simulink model "Studienarbeit"  (R2020a)
settings: Solver=VariableStepAuto  StartTime=0.0  StopTime=300  FixedStep=0.1  RelTol=1e-3
values from neighbouring files (symbols this model uses):
  driver_I = 0.1    [Buses_.mat]    (also in helperACCSetUp.m)
  driver_P = 0.2    [Buses_.mat]    (also in helperACCSetUp.m)
  initial_lane = 0    [helperACCSetUp.m]
  lr = 1.6    [Buses_.mat]    (also in helperACCSetUp.m)
  m = 1575    [Buses_.mat]    (also in helperACCSetUp.m)
  tau = 0.5    [Buses_.mat]    (also in helperACCSetUp.m)
  velocity_left_lane_max = 28    [Buses_.mat]    (also in helperManeuverSetUp.m)
  velocity_right_lane_max = 20    [Buses_.mat]    (also in helperManeuverSetUp.m)
  velocity_vehicle_B = 10    [Buses_.mat]    (also in helperManeuverSetUp.m)
  yawerr_gain = 2    [Buses_.mat]    (also in helperACCSetUp.m)
undefined symbols (not defined in the file or in its folder): Curvature, CurvatureDerivative, driving, HeadingAngle, LateralOffset, Left, Right, Strength
libraries: drivingscenarioandsensors x3, simulink x1, autolibshared x1
(part 1 of 2)
Description:
  | This model combines lane keeping assist and adaptive cruise control to achieve overtaking maneuver
settings Model: Creator=JiangHeng  LastModifiedBy=JiangHeng

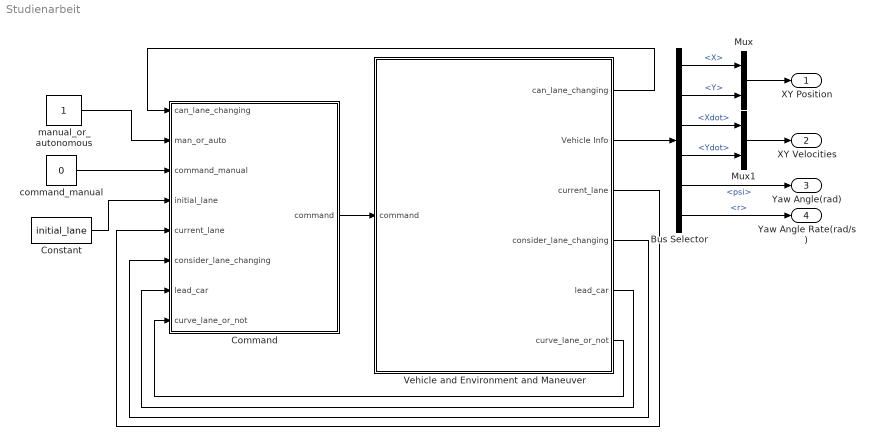
== system Studienarbeit ==
  Bus Selector : BusSelector  OutputSignals=InertFrm.FrntAxl.Disp.X,InertFrm.FrntAxl.Disp.Y,InertFrm.FrntAxl.Vel.Xdot,InertFrm.FrntAxl.Vel.Ydot,InertFrm.Cg.Ang.psi,BdyFrm.Cg.AngVel.r
  Command : Stateflow chart  TreatAsAtomicUnit=on
      settings: PortSchema="{\"entries\":[{\"content\":{\"sides\":[{\"content\":{\"connectorIds\":[\"In1\",\"In2\",\"In5\",\"In6\",\"In7\",\"In3\",\"In4\",\"In8\"]},\"type\":\"ConnectorPlacement.EquallySpacedRectSide\",\"uuid\":\"73bcf0fb-eeaf-43f1-b597-f0232c0f98c1\"},{\"content\":{\"connectorIds\":[\"Out1\"],\"side\":\"RIGHT\"},\"type\":\"ConnectorPlacement.EquallySpacedRectSide\",\"uuid\":\"41fc5fcb-a6b0-4783-b0ea-910aa524831f\"},{\"content\":{\"connectorIds\":[],\"side\":\"TOP\"},\"type\":\"ConnectorPlacement.EquallySpacedRectSide\",\"uuid\":\"53b92c3f-3309-4abb-be29-ad8d06433ab2\"},{\"content\":{\"connectorIds\":[],\"side\":\"BOTTOM\"},\"type\":\"ConnectorPlacement.EquallySpacedRectSide\",\"uuid\":\"12113223-5d1b-44a7-bb57-d0482123bc44\"}]},\"type\":\"ConnectorPlacement.EquallySpacedConnector\",\"uuid\":\"d001029e-52d5-4d88-96e8-8c112339464d\"}],\"packageUris\":[\"http://schema.mathworks.com/mf0/Connector/19700101\"],\"version\":\"1.0\"}"
  Constant : Constant  Value=initial_lane
  Mux : Mux  Inputs=2
  Mux1 : Mux  Inputs=2
  Vehicle and Environment and Maneuver : Subsystem
  command_manual : Constant  Value=0
  manual_or_autonomous : Constant
  XY Position : Outport
  XY Velocities : Outport  Port=2
  Yaw Angle(rad) : Outport  Port=3
  Yaw Angle Rate(rad/s) : Outport  Port=4
  wires:
  Command/1(command) -> Vehicle and Environment and Maneuver/1(command)
  Bus Selector/2 -> Mux/2  "<Y>"
  Bus Selector/1 -> Mux/1  "<X>"
  Bus Selector/3 -> Mux1/1  "<Xdot>"
  Bus Selector/4 -> Mux1/2  "<Ydot>"
  Mux/1 -> XY Position/1
  Bus Selector/5 -> Yaw Angle(rad)/1  "<psi>"
  Bus Selector/6 -> Yaw Angle Rate(rad/s)/1  "<r>"
  Vehicle and Environment and Maneuver/2(Vehicle Info) -> Bus Selector/1
  Mux1/1 -> XY Velocities/1
  Vehicle and Environment and Maneuver/1(can_lane_changing) -> Command/1(can_lane_changing)
  Vehicle and Environment and Maneuver/3(current_lane) -> Command/7(current_lane)
  Vehicle and Environment and Maneuver/4(consider_lane_changing) -> Command/3(consider_lane_changing)
  Vehicle and Environment and Maneuver/5(lead_car) -> Command/4(lead_car)
  Constant/1 -> Command/6(initial_lane)
  manual_or_autonomous/1 -> Command/2(man_or_auto)
  Vehicle and Environment and Maneuver/6(curve_lane_or_not) -> Command/8(curve_lane_or_not)
  command_manual/1 -> Command/5(command_manual)

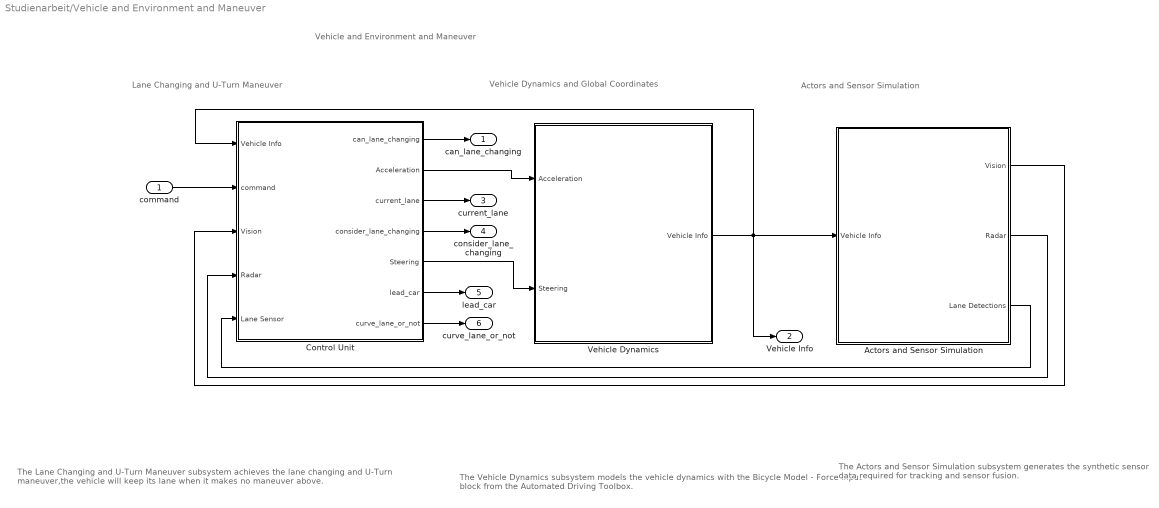
== system Studienarbeit/Vehicle and Environment and Maneuver ==
  note: Lane Changing and U-Turn Maneuver
  note: The Vehicle Dynamics subsystem models
      | the vehicle dynamics with the Bicycle
      | Model - Force Input block from the Automated
      | Driving Toolbox.
  note: The Actors and Sensor Simulation
      | subsystem generates the synthetic
      | sensor data required for tracking
      | and sensor fusion.
  note: Actors and Sensor Simulation
  note: Vehicle and Environment and Maneuver
  note: Vehicle Dynamics and Global Coordinates
  note: The Lane Changing and U-Turn Maneuver subsystem
      | achieves the lane changing and U-Turn maneuver,the
      | vehicle will keep its lane when it makes no maneuver
      | above.
  command : Inport
  Actors and Sensor Simulation : Subsystem
  Control Unit : Subsystem
  Vehicle Dynamics : Subsystem  VariantControl=Variant2
  can_lane_changing : Outport
  Vehicle Info : Outport  Port=2
  current_lane : Outport  Port=3
  consider_lane_changing : Outport  Port=4
  lead_car : Outport  Port=5
  curve_lane_or_not : Outport  Port=6
  wires:
  Actors and Sensor Simulation/1(Vision) -> Control Unit/3(Vision)
  Actors and Sensor Simulation/2(Radar) -> Control Unit/4(Radar)
  Control Unit/2(Acceleration) -> Vehicle Dynamics/1(Acceleration)
  Control Unit/5(Steering) -> Vehicle Dynamics/2(Steering)
  Vehicle Dynamics/1(Vehicle Info) -> Control Unit/1(Vehicle Info), Vehicle Info/1, Actors and Sensor Simulation/1(Vehicle Info)
  Actors and Sensor Simulation/3(Lane Detections) -> Control Unit/5(Lane Sensor)
  Control Unit/1(can_lane_changing) -> can_lane_changing/1
  Control Unit/3(current_lane) -> current_lane/1
  Control Unit/4(consider_lane_changing) -> consider_lane_changing/1
  Control Unit/6(lead_car) -> lead_car/1
  Control Unit/7(curve_lane_or_not) -> curve_lane_or_not/1
  command/1 -> Control Unit/2(command)

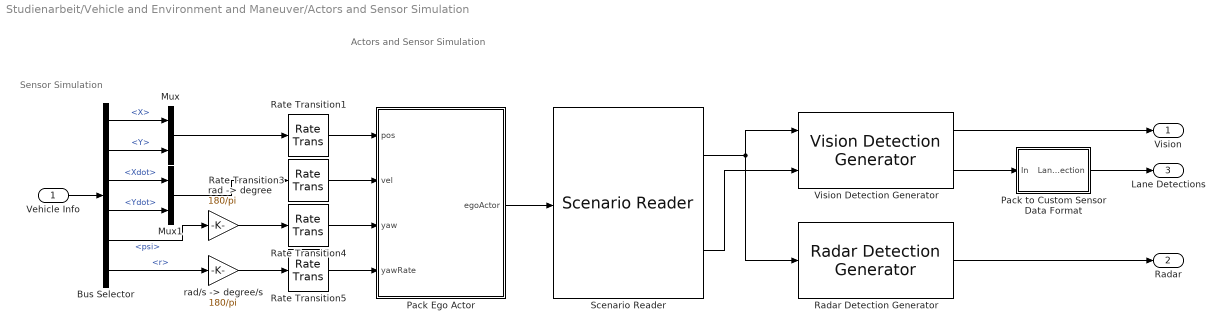
== system Studienarbeit/Vehicle and Environment and Maneuver/Actors and Sensor Simulation ==
  note: Sensor Simulation
  note: Actors and Sensor Simulation
  Vehicle Info : Inport
  Bus Selector : BusSelector  OutputSignals=InertFrm.FrntAxl.Disp.X,InertFrm.FrntAxl.Disp.Y,InertFrm.FrntAxl.Vel.Xdot,InertFrm.FrntAxl.Vel.Ydot,InertFrm.Cg.Ang.psi,BdyFrm.Cg.AngVel.r
  Mux : Mux  Inputs=2
  Mux1 : Mux  Inputs=2
  Pack Ego Actor : MATLAB Function  TreatAsAtomicUnit=on
  Pack to Custom Sensor Data Format : Subsystem
  Radar Detection Generator : drivingscenarioandsensors/Radar Detection Generator  SensorIndex=2  UpdateInterval=0.1  SensorLocation=[ 3.7, 0 ]  Height=0.2  Yaw=0  Pitch=0  Roll=0  BusNameSource=Property  BusName=BusRadar  MaxNumDetectionsSource=Property  MaxNumDetections=50  DetectionCoordinates=Ego Cartesian  SimulateUsing=Interpreted execution  AzimuthResolution=4  ElevationResolution=10  RangeResolution=2.5  RangeRateResolution=0.5  AzimuthBiasFraction=0.1  ElevationBiasFraction=0.1  RangeBiasFraction=0.05  RangeRateBiasFraction=0.05  FieldOfView=[ 20, 5 ]  MaxRange=174  RangeRateLimits=[ -100, 100 ]  DetectionProbability=0.9  FalseAlarmRate=1e-6  ReferenceRange=100  ReferenceRCS=0  HasElevation=off  HasRangeRate=on  HasNoise=on  HasFalseAlarms=on  HasOcclusion=on  InitialSeedSource=Repeatable  InitialSeed=0  UsedSeed=driving.internal.SimulinkUtilities.seedManager(gcb)  ActorProfilesSource=Parameters  ActorProfilesParameters=driving.internal.ActorProfilesRadarParameters  ActorProfilesExpression=struct( 'ClassID', 0, 'Length', 4.7, 'Width', 1.8, 'Height', 1.4, 'OriginOffset', [ -1.35, 0, 0 ], 'RCSPattern', [ 10, 10; 10, 10 ], 'RCSAzimuthAngles', [ -180, 180 ], 'RCSElevationAngles', [ -90, 90 ] )
      settings: SourceProductBaseCode=DR
  Rate Transition{1,3..5} (4 alike) : RateTransition  OutPortSampleTime=Ts
  Scenario Reader : drivingscenarioandsensors/Scenario Reader  ScenarioSource=From file  ScenarioFileName=.\LaneChange.mat  ScenarioVariableName=scenario  OutputCoordinateSystem=Vehicle coordinates  EgoVehicleSource=Input port  OrientVehiclesOnRoad=off  EgoVehicleActorID=1  OutputEgoVehiclePose=off  SampleTime=0.1  LaneBoundaryOutput=Ego vehicle lane boundaries  LaneBoundaryDistance=0:0.5:9.5  LaneBoundaryLocation=Center of lane markings  BusNameSource=Auto  BusName=BusActors  BusName2Source=Auto  BusName2=BusVision1  BusName3Source=Auto  BusName3=BusEgoActor  ShowCoordinateLabels=on  SimulateUsing=Interpreted execution
  Vision Detection Generator : drivingscenarioandsensors/Vision Detection Generator  SensorIndex=1  DetectorOutput=Lanes and objects  UpdateInterval=0.1  LaneUpdateInterval=0.1  SensorLocation=[ 2.1, 0 ]  Height=1.1  Yaw=0  Pitch=1  Roll=0  BusNameSource=Property  BusName=BusVision  BusName2Source=Property  BusName2=BusVision1  MaxNumDetectionsSource=Property  MaxNumDetections=20  MaxNumLanesSource=Property  MaxNumLanes=2  DetectionCoordinates=Ego Cartesian  SimulateUsing=Interpreted execution  MaxRange=150  BoundingBoxAccuracy=5  ProcessNoiseIntensity=5  MaxSpeed=50  MaxAllowedOcclusion=0.5  MinObjectImageSize=[ 15, 15 ]  DetectionProbability=0.9  FalsePositivesPerImage=0.1  MinLaneImageSize=[ 20, 5 ]  LaneBoundaryAccuracy=3  HasNoise=on  InitialSeedSource=Repeatable  InitialSeed=0  UsedSeed=driving.internal.SimulinkUtilities.seedManager(gcb)  ActorProfilesSource=Parameters  ActorProfilesParameters=driving.internal.ActorProfilesParameters  ActorProfilesExpression=struct( 'ClassID', 0, 'Length', 4.7, 'Width', 1.8, 'Height', 1.4, 'OriginOffset', [ -1.35, 0, 0 ] )  Intrinsics=driving.internal.cameraIntrinsics
  "rad -> degree" : Gain  Gain=180/pi
  "rad/s -> degree/s" : Gain  Gain=180/pi
  Vision : Outport  VectorParamsAs1DForOutWhenUnconnected=off
  Radar : Outport  Port=2  VectorParamsAs1DForOutWhenUnconnected=off
  Lane Detections : Outport  Port=3
  wires:
  Scenario Reader/1 -> Radar Detection Generator/1, Vision Detection Generator/1
  Vision Detection Generator/1 -> Vision/1
  Pack Ego Actor/1(egoActor) -> Scenario Reader/1
  Radar Detection Generator/1 -> Radar/1
  Rate Transition1/1 -> Pack Ego Actor/1(pos)
  Rate Transition3/1 -> Pack Ego Actor/2(vel)
  Rate Transition5/1 -> Pack Ego Actor/4(yawRate)
  Rate Transition4/1 -> Pack Ego Actor/3(yaw)
  Bus Selector/4 -> Mux1/2  "<Ydot>"
  Mux/1 -> Rate Transition1/1
  Bus Selector/2 -> Mux/2  "<Y>"
  Bus Selector/3 -> Mux1/1  "<Xdot>"
  Bus Selector/1 -> Mux/1  "<X>"
  Vehicle Info/1 -> Bus Selector/1
  "rad/s -> degree/s"/1 -> Rate Transition5/1
  "rad -> degree"/1 -> Rate Transition4/1
  Bus Selector/5 -> "rad -> degree"/1  "<psi>"
  Bus Selector/6 -> "rad/s -> degree/s"/1  "<r>"
  Scenario Reader/2 -> Vision Detection Generator/2
  Vision Detection Generator/2 -> Pack to Custom Sensor Data Format/1(In)
  Pack to Custom Sensor Data Format/1(Lane Detection) -> Lane Detections/1
  Mux1/1 -> Rate Transition3/1

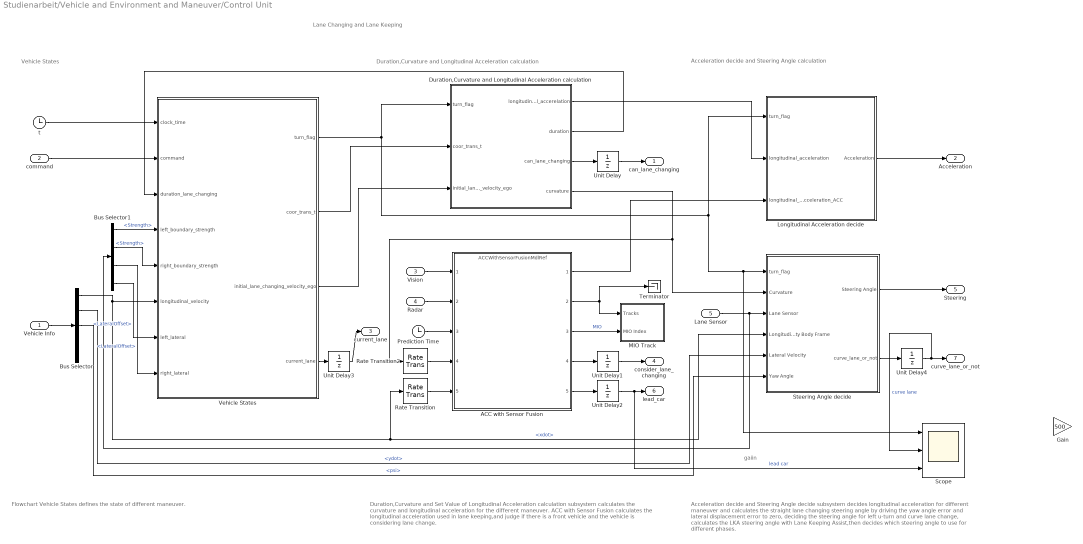
== system Studienarbeit/Vehicle and Environment and Maneuver/Control Unit ==
  note: gaiin
  note: Duration,Curvature and Longitudinal Acceleration calculation
  note: Acceleration decide and Steering Angle decide subsystem
      | decides longitudinal acceleration for different maneuver and
      | calculates the straight lane changing steering angle by driving
      | the yaw angle error and lateral displacement error to zero,
      | deciding the steering angle for left u-turn and curve lane change,
      | calculates the LKA steering angle with Lane Keeping Assist,then
      | decides which steering angle to use for different phases.
  note: Duration,Curvature and Set Value of Longitudinal
      | Acceleration calculation subsystem calculates the
      | curvature and longitudinal acceleration for the different
      | maneuver.
      | ACC with Sensor Fusion calculates the longitudinal
      | acceleration used in lane keeping,and judge if there is a
      | front vehicle and the vehicle is considering lane change.
  note: Acceleration decide and Steering Angle calculation
  note: Vehicle States
  note: Flowchart Vehicle States defines the state of different maneuver.
  note: Lane Changing and Lane Keeping
  Vehicle Info : Inport
  command : Inport  Port=2
  Vision : Inport  Port=3
  Radar : Inport  Port=4
  Lane Sensor : Inport  Port=5
  ACC with Sensor Fusion : ModelReference  ModelNameDialog=ACCWithSensorFusionMdlRef.slx  SimulationMode=Normal  CodeInterface=Top model  ModelReferenceVersion=1.495
  Bus Selector : BusSelector  OutputSignals=BdyFrm.FrntAxl.Vel.xdot,BdyFrm.FrntAxl.Vel.ydot,InertFrm.Cg.Ang.psi,InertFrm.FrntAxl.Disp.X,InertFrm.FrntAxl.Disp.Y
  Bus Selector1 : BusSelector  OutputSignals=Left.Strength,Right.Strength,Right.LateralOffset,Left.LateralOffset
  Duration,Curvature and Longitudinal Acceleration calculation : Subsystem
  Gain : Gain  Gain=500
  Longitudinal Acceleration decide : Subsystem
  MIO Track : Subsystem
  Prediction Time : Clock
  Rate Transition : RateTransition  OutPortSampleTime=Ts
  Rate Transition2 : RateTransition  OutPortSampleTime=Ts
  Scope : Scope  NumInputPorts=3
  Steering Angle decide : Subsystem
  Terminator : Terminator
  Unit Delay{,1..4} (5 alike) : UnitDelay  SampleTime=-1  HasFrameUpgradeWarning=on
  Vehicle States : Stateflow chart  TreatAsAtomicUnit=on
      settings: PortSchema="{\"entries\":[{\"content\":{\"sides\":[{\"content\":{\"connectorIds\":[\"In2\",\"In1\",\"In3\",\"In4\",\"In5\",\"In6\",\"In7\",\"In8\"]},\"type\":\"ConnectorPlacement.EquallySpacedRectSide\",\"uuid\":\"633906ca-579d-4042-9cc9-7aca433b340e\"},{\"content\":{\"connectorIds\":[\"Out1\",\"Out2\",\"Out3\",\"Out4\"],\"side\":\"RIGHT\"},\"type\":\"ConnectorPlacement.EquallySpacedRectSide\",\"uuid\":\"b2f4b13f-832c-4f85-a2c3-5544fdd2b38b\"},{\"content\":{\"connectorIds\":[],\"side\":\"TOP\"},\"type\":\"ConnectorPlacement.EquallySpacedRectSide\",\"uuid\":\"a13a6fde-8974-48e1-9856-53eff330f07d\"}]},\"type\":\"ConnectorPlacement.EquallySpacedConnector\",\"uuid\":\"3aa8cc94-316d-4e92-871e-4708a17b4e4c\"}],\"packageUris\":[\"http://schema.mathworks.com/mf0/Connector/19700101\"],\"version\":\"1.0\"}"
  t : Clock
  can_lane_changing : Outport
  Acceleration : Outport  Port=2
  current_lane : Outport  Port=3
  consider_lane_changing : Outport  Port=4
  Steering : Outport  Port=5
  lead_car : Outport  Port=6
  curve_lane_or_not : Outport  Port=7
  wires:
  command/1 -> Vehicle States/1(command)
  ACC with Sensor Fusion/1 -> Longitudinal Acceleration decide/3(longitudinal_acceleration_ACC)
  Vehicle States/2(coor_trans_t) -> Duration,Curvature and Longitudinal Acceleration calculation/2(coor_trans_t)
  Longitudinal Acceleration decide/1(Acceleration) -> Acceleration/1
  Bus Selector/2 -> Steering Angle decide/5(Lateral Velocity)  "<ydot>"
  ACC with Sensor Fusion/3 -> MIO Track/2(MIO Index)  "MIO"
  ACC with Sensor Fusion/2 -> Terminator/1, MIO Track/1(Tracks)
  Rate Transition2/1 -> ACC with Sensor Fusion/4
  Rate Transition/1 -> ACC with Sensor Fusion/5
  t/1 -> Vehicle States/2(clock_time)
  Radar/1 -> ACC with Sensor Fusion/2
  Vision/1 -> ACC with Sensor Fusion/1
  Vehicle States/3(initial_lane_changing_velocity_ego) -> Duration,Curvature and Longitudinal Acceleration calculation/3(initial_lane_changing_velocity_ego)
  Duration,Curvature and Longitudinal Acceleration calculation/1(longitudinal_accerelation) -> Longitudinal Acceleration decide/2(longitudinal_acceleration)
  Vehicle Info/1 -> Bus Selector/1
  Bus Selector/1 -> Rate Transition/1, Steering Angle decide/4(Longitudinal Velocity Body Frame), Vehicle States/6(longitudinal_velocity)  "<xdot>"
  Steering Angle decide/1(Steering Angle) -> Steering/1
  Duration,Curvature and Longitudinal Acceleration calculation/3(can_lane_changing) -> Unit Delay/1
  Vehicle States/4(current_lane) -> Unit Delay3/1
  Unit Delay/1 -> can_lane_changing/1
  ACC with Sensor Fusion/4 -> Unit Delay1/1
  ACC with Sensor Fusion/5 -> Unit Delay2/1
  Unit Delay1/1 -> consider_lane_changing/1
  Unit Delay2/1 -> Scope/3, lead_car/1  "lead car"
  Unit Delay3/1 -> current_lane/1
  Steering Angle decide/2(curve_lane_or_not) -> Unit Delay4/1
  Unit Delay4/1 -> Scope/2, curve_lane_or_not/1  "curve lane"
  Bus Selector/3 -> Steering Angle decide/6(Yaw Angle)  "<psi>"
  Lane Sensor/1 -> Steering Angle decide/3(Lane Sensor), Bus Selector1/1
  Vehicle States/1(turn_flag) -> Duration,Curvature and Longitudinal Acceleration calculation/1(turn_flag), Scope/1, Steering Angle decide/1(turn_flag), Longitudinal Acceleration decide/1(turn_flag)
  Duration,Curvature and Longitudinal Acceleration calculation/2(duration) -> Vehicle States/3(duration_lane_changing)
  Bus Selector1/3 -> Vehicle States/8(right_lateral)  "<LateralOffset>"
  Bus Selector1/4 -> Vehicle States/7(left_lateral)  "<LateralOffset>"
  Bus Selector1/1 -> Vehicle States/4(left_boundary_strength)  "<Strength>"
  Bus Selector1/2 -> Vehicle States/5(right_boundary_strength)  "<Strength>"
  Prediction Time/1 -> ACC with Sensor Fusion/3
  Duration,Curvature and Longitudinal Acceleration calculation/4(curvature) -> Steering Angle decide/2(Curvature), Rate Transition2/1

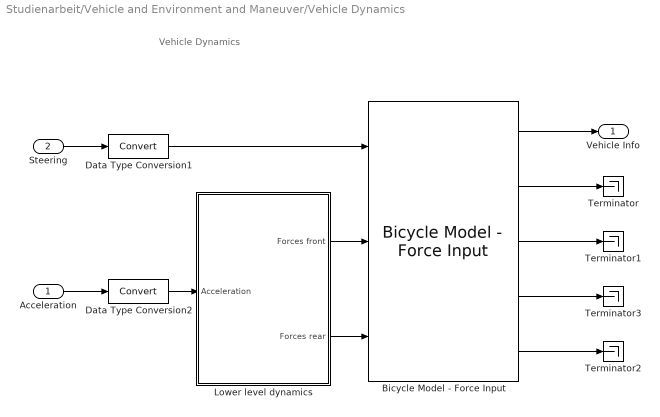
== system Studienarbeit/Vehicle and Environment and Maneuver/Vehicle Dynamics ==
  note: Vehicle Dynamics
  Acceleration : Inport  Unit=m/s^2
  Steering : Inport  Port=2  Unit=rad
  Bicycle Model - Force Input : autolibshared/Bicycle Model - Force Input  trackMode=Single (bicycle)  inputMode=External longitudinal forces  frontSteerMode=on  rearSteerMode=off  windMode=off  muMode=off  extFMode=off  extMMode=off  aMode=3  NF=2  NR=2  m=m  a=lf  b=lr  h=0.35  X_o=x0_ego  xdot_o=v0_ego  CalphaMode=off  sigmaMode=on  w=[1.4,1.4]  Cy_f=Cf  Cy_r=Cr  sigma_f=.1  sigma_r=.1  alpha_f_brk=[-.1 .1]  Cy_f_data=[-9e3 9e3]  alpha_r_brk=[-.1 .1]  Cy_r_data=[-9e3 9e3]  Y_o=y0_ego  ydot_o=0  Izz=Iz  psi_o=0  r_o=0  Af=0  Cd=.3  Cl=.1  Cpm=.1  beta_w=[0:0.01:0.3]  Cs=[0:0.03:0.9]  Cym=[0:0.01:0.3]  Pabs=101325  Tair=273  g=9.81  mu=1  xdot_tol=.01  Fznom=5000  Fxtire_sat=1e6  Fytire_sat=1e6  longOff=0  latOff=0  vertOff=0
      settings: SourceProductBaseCode=PW,MT,VE,VP
  Data Type Conversion1 : DataTypeConversion
  Data Type Conversion2 : DataTypeConversion
  Lower level dynamics : Subsystem
  Terminator{,1..3} (4 alike) : Terminator
  Vehicle Info : Outport  Unit=m  VectorParamsAs1DForOutWhenUnconnected=off
  wires:
  Data Type Conversion2/1 -> Lower level dynamics/1(Acceleration)
  Acceleration/1 -> Data Type Conversion2/1
  Steering/1 -> Data Type Conversion1/1
  Bicycle Model - Force Input/4 -> Terminator3/1
  Bicycle Model - Force Input/5 -> Terminator2/1
  Data Type Conversion1/1 -> Bicycle Model - Force Input/1
  Bicycle Model - Force Input/3 -> Terminator1/1
  Bicycle Model - Force Input/1 -> Vehicle Info/1
  Bicycle Model - Force Input/2 -> Terminator/1
  Lower level dynamics/1(Forces front) -> Bicycle Model - Force Input/2
  Lower level dynamics/2(Forces rear) -> Bicycle Model - Force Input/3

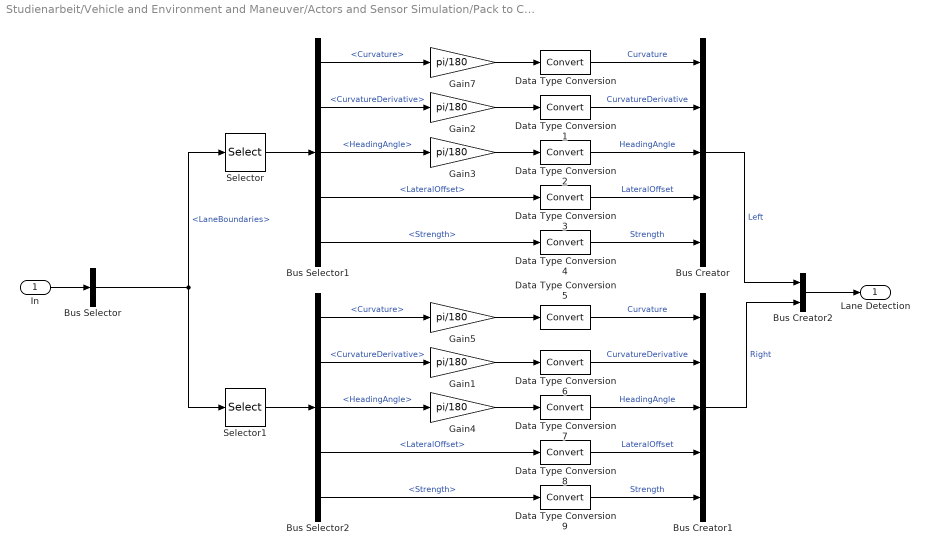
== system Studienarbeit/Vehicle and Environment and Maneuver/Actors and Sensor Simulation/Pack to Custom Sensor Data Format ==
  In : Inport
  Bus Creator : BusCreator  Inputs=Curvature,CurvatureDerivative,HeadingAngle,LateralOffset,Strength  OutDataTypeStr=Bus: LaneSensorBoundaries
  Bus Creator1 : BusCreator  Inputs=Curvature,CurvatureDerivative,HeadingAngle,LateralOffset,Strength  OutDataTypeStr=Bus: LaneSensorBoundaries
  Bus Creator2 : BusCreator  Inputs=Left,Right  OutDataTypeStr=Bus: LaneSensor
  Bus Selector : BusSelector  OutputSignals=LaneBoundaries
  Bus Selector1 : BusSelector  OutputSignals=Curvature,CurvatureDerivative,HeadingAngle,LateralOffset,Strength
  Bus Selector2 : BusSelector  OutputSignals=Curvature,CurvatureDerivative,HeadingAngle,LateralOffset,Strength
  Data Type Conversion{,1..9} (10 alike) : DataTypeConversion
  Gain{1..5,7} (6 alike) : Gain  Gain=pi/180
  Selector : Selector  InputPortWidth=2  IndexOptions=Index vector (dialog)  Indices=1  OutputSizes=1
  Selector1 : Selector  InputPortWidth=2  IndexOptions=Index vector (dialog)  Indices=2  OutputSizes=1
  Lane Detection : Outport  VectorParamsAs1DForOutWhenUnconnected=off
  wires:
  In/1 -> Bus Selector/1
  Bus Selector/1 -> Selector/1, Selector1/1  "<LaneBoundaries>"
  Selector/1 -> Bus Selector1/1
  Bus Selector1/2 -> Gain2/1  "<CurvatureDerivative>"
  Bus Selector1/1 -> Gain7/1  "<Curvature>"
  Bus Selector1/3 -> Gain3/1  "<HeadingAngle>"
  Gain7/1 -> Data Type Conversion/1
  Gain2/1 -> Data Type Conversion1/1
  Gain3/1 -> Data Type Conversion2/1
  Bus Selector1/4 -> Data Type Conversion3/1  "<LateralOffset>"
  Bus Selector1/5 -> Data Type Conversion4/1  "<Strength>"
  Data Type Conversion/1 -> Bus Creator/1  "Curvature"
  Data Type Conversion1/1 -> Bus Creator/2  "CurvatureDerivative"
  Data Type Conversion2/1 -> Bus Creator/3  "HeadingAngle"
  Data Type Conversion3/1 -> Bus Creator/4  "LateralOffset"
  Data Type Conversion4/1 -> Bus Creator/5  "Strength"
  Data Type Conversion9/1 -> Bus Creator1/5  "Strength"
  Data Type Conversion6/1 -> Bus Creator1/2  "CurvatureDerivative"
  Data Type Conversion7/1 -> Bus Creator1/3  "HeadingAngle"
  Data Type Conversion8/1 -> Bus Creator1/4  "LateralOffset"
  Data Type Conversion5/1 -> Bus Creator1/1  "Curvature"
  Bus Selector2/1 -> Gain5/1  "<Curvature>"
  Selector1/1 -> Bus Selector2/1
  Bus Selector2/4 -> Data Type Conversion8/1  "<LateralOffset>"
  Bus Selector2/5 -> Data Type Conversion9/1  "<Strength>"
  Bus Selector2/2 -> Gain1/1  "<CurvatureDerivative>"
  Gain4/1 -> Data Type Conversion7/1
  Gain5/1 -> Data Type Conversion5/1
  Gain1/1 -> Data Type Conversion6/1
  Bus Selector2/3 -> Gain4/1  "<HeadingAngle>"
  Bus Creator2/1 -> Lane Detection/1
  Bus Creator/1 -> Bus Creator2/1  "Left"
  Bus Creator1/1 -> Bus Creator2/2  "Right"

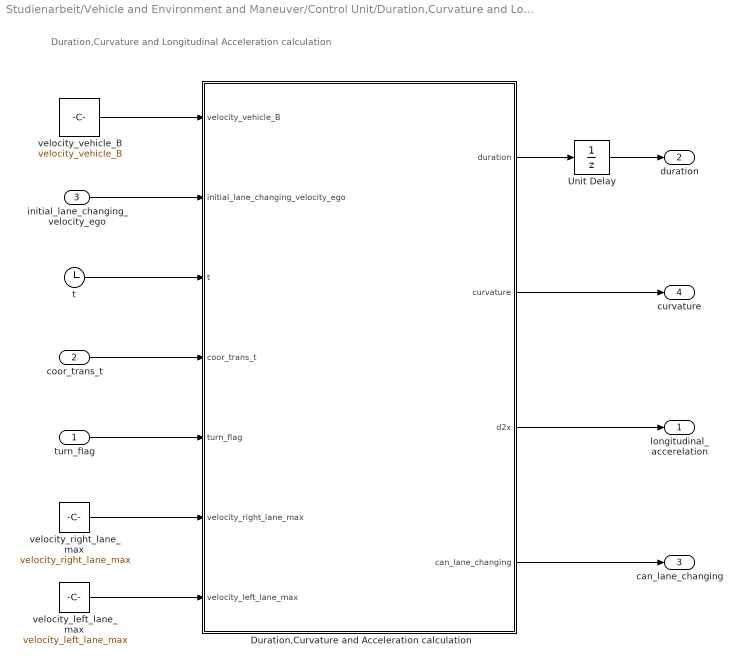
== system Studienarbeit/Vehicle and Environment and Maneuver/Control Unit/Duration,Curvature and Longitudinal Acceleration calculation ==
  note: Duration,Curvature and Longitudinal Acceleration calculation
  turn_flag : Inport
  coor_trans_t : Inport  Port=2
  initial_lane_changing_velocity_ego : Inport  Port=3
  Duration,Curvature and Acceleration calculation : MATLAB Function  TreatAsAtomicUnit=on
  Unit Delay : UnitDelay  SampleTime=-1  HasFrameUpgradeWarning=on
  t : Clock
  velocity_left_lane_max : Constant  Value=velocity_left_lane_max
  velocity_right_lane_max : Constant  Value=velocity_right_lane_max
  velocity_vehicle_B : Constant  Value=velocity_vehicle_B
  longitudinal_accerelation : Outport
  duration : Outport  Port=2
  can_lane_changing : Outport  Port=3
  curvature : Outport  Port=4
  wires:
  coor_trans_t/1 -> Duration,Curvature and Acceleration calculation/4(coor_trans_t)
  initial_lane_changing_velocity_ego/1 -> Duration,Curvature and Acceleration calculation/2(initial_lane_changing_velocity_ego)
  velocity_vehicle_B/1 -> Duration,Curvature and Acceleration calculation/1(velocity_vehicle_B)
  t/1 -> Duration,Curvature and Acceleration calculation/3(t)
  turn_flag/1 -> Duration,Curvature and Acceleration calculation/5(turn_flag)
  velocity_right_lane_max/1 -> Duration,Curvature and Acceleration calculation/6(velocity_right_lane_max)
  velocity_left_lane_max/1 -> Duration,Curvature and Acceleration calculation/7(velocity_left_lane_max)
  Duration,Curvature and Acceleration calculation/4(can_lane_changing) -> can_lane_changing/1
  Unit Delay/1 -> duration/1
  Duration,Curvature and Acceleration calculation/1(duration) -> Unit Delay/1
  Duration,Curvature and Acceleration calculation/3(d2x) -> longitudinal_accerelation/1
  Duration,Curvature and Acceleration calculation/2(curvature) -> curvature/1

== system Studienarbeit/Vehicle and Environment and Maneuver/Control Unit/Longitudinal Acceleration decide ==
  note: This subsystem's output is longitudinal acceleration.
      | Switch determine that which acceleration (from ACC or from calculation)is used for different phases(lane changing,U-Turn or go straight)with turn_flag:
      | turn_flag = 1,2,lane changing
      | turn_flag = 0,go straight
      | turn_flag = 3,4,curve lane changing
      | turn_flag =5,6,7,8,left U-Turn
  note: Longitudinal Acceleration decide
  turn_flag : Inport
  longitudinal_acceleration : Inport  Port=2
  longitudinal_acceleration_ACC : Inport  Port=3
  Switch : Switch  Criteria=u2 > Threshold
  Acceleration : Outport
  wires:
  longitudinal_acceleration/1 -> Switch/1
  turn_flag/1 -> Switch/2
  longitudinal_acceleration_ACC/1 -> Switch/3
  Switch/1 -> Acceleration/1

== system Studienarbeit/Vehicle and Environment and Maneuver/Control Unit/MIO Track ==
  note: Extract MIO and Package as Track for Visualization in Birds Eye Scope
  Tracks : Inport
  MIO Index : Inport  Port=2
  Pack MIO Track : MATLAB Function  TreatAsAtomicUnit=on
  Terminator : Terminator
  wires:
  Pack MIO Track/1(mioTrack) -> Terminator/1  "mio_track"
  Tracks/1 -> Pack MIO Track/1(tracks)
  MIO Index/1 -> Pack MIO Track/2(mioTrackIndex)

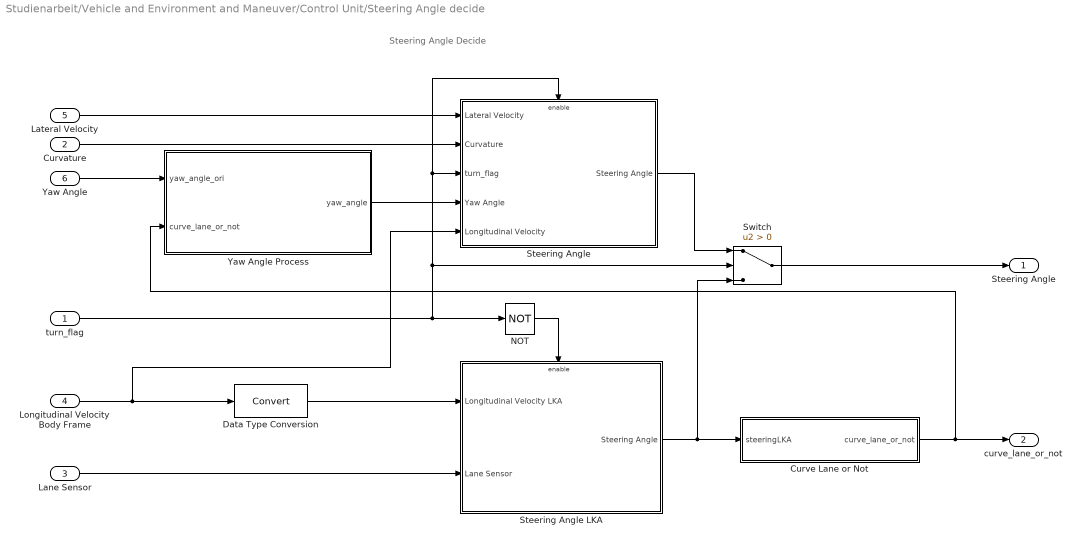
== system Studienarbeit/Vehicle and Environment and Maneuver/Control Unit/Steering Angle decide ==
  note: Steering Angle Decide
  turn_flag : Inport
  Curvature : Inport  Port=2
  Lane Sensor : Inport  Port=3
  Longitudinal Velocity Body Frame : Inport  Port=4
  Lateral Velocity : Inport  Port=5
  Yaw Angle : Inport  Port=6
  Curve Lane or Not : MATLAB Function  TreatAsAtomicUnit=on
  Data Type Conversion : DataTypeConversion
  NOT : Logic  Operator=NOT  IconShape=distinctive  AllPortsSameDT=off  OutDataTypeStr=boolean
  "Steering Angle " : Subsystem  TreatAsAtomicUnit=on
  Steering Angle LKA : Subsystem  TreatAsAtomicUnit=on
  Switch : Switch  Criteria=u2 > Threshold
  Yaw Angle Process : MATLAB Function  TreatAsAtomicUnit=on
  Steering Angle : Outport
  curve_lane_or_not : Outport  Port=2
  wires:
  Switch/1 -> Steering Angle/1
  "Steering Angle "/1(Steering Angle) -> Switch/1
  Steering Angle LKA/1(Steering Angle) -> Switch/3, Curve Lane or Not/1(steeringLKA)
  turn_flag/1 -> "Steering Angle "/Enable, "Steering Angle "/3(turn_flag), Switch/2, NOT/1
  NOT/1 -> Steering Angle LKA/Enable
  Lateral Velocity/1 -> "Steering Angle "/1(Lateral Velocity)
  Curvature/1 -> "Steering Angle "/2(Curvature)
  Lane Sensor/1 -> Steering Angle LKA/2(Lane Sensor)
  Yaw Angle Process/1(yaw_angle) -> "Steering Angle "/4(Yaw Angle)
  Curve Lane or Not/1(curve_lane_or_not) -> curve_lane_or_not/1, Yaw Angle Process/2(curve_lane_or_not)
  Longitudinal Velocity Body Frame/1 -> Data Type Conversion/1, "Steering Angle "/5(Longitudinal Velocity)
  Data Type Conversion/1 -> Steering Angle LKA/1(Longitudinal Velocity LKA)
  Yaw Angle/1 -> Yaw Angle Process/1(yaw_angle_ori)

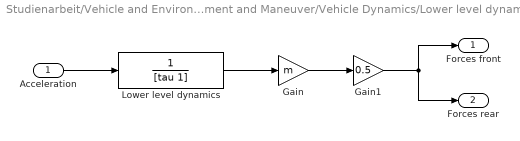
== system Studienarbeit/Vehicle and Environment and Maneuver/Vehicle Dynamics/Lower level dynamics ==
  Acceleration : Inport
  Gain : Gain  Gain=m
  Gain1 : Gain  Gain=0.5
  Lower level dynamics : TransferFcn  Denominator=[tau 1]
  Forces front : Outport  VectorParamsAs1DForOutWhenUnconnected=off
  Forces rear : Outport  Port=2  VectorParamsAs1DForOutWhenUnconnected=off
  wires:
  Gain/1 -> Gain1/1
  Gain1/1 -> Forces front/1, Forces rear/1
  Lower level dynamics/1 -> Gain/1
  Acceleration/1 -> Lower level dynamics/1

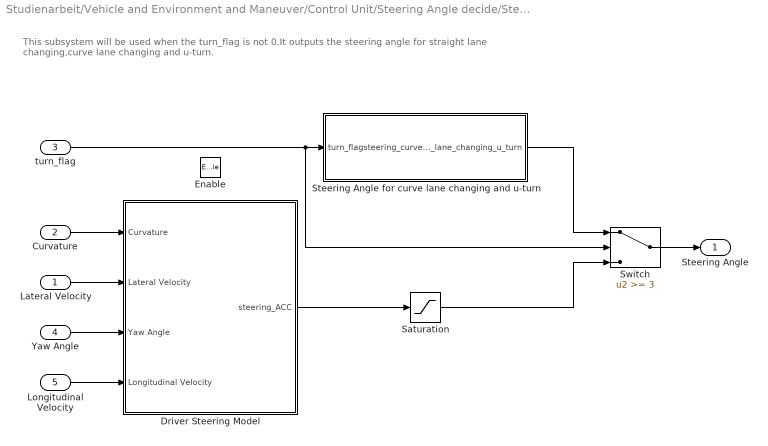
== system Studienarbeit/Vehicle and Environment and Maneuver/Control Unit/Steering Angle decide/Steering Angle  ==
  note: This subsystem will be used when the turn_flag is not 0.It outputs the steering angle for
      | straight lane changing,curve lane changing and u-turn.
  Lateral Velocity : Inport
  Curvature : Inport  Port=2
  turn_flag : Inport  Port=3
  Yaw Angle : Inport  Port=4
  Longitudinal Velocity : Inport  Port=5
  Enable : EnablePort
  Driver Steering Model : Subsystem
  Saturation : Saturate
  Steering Angle for curve lane changing and u-turn : MATLAB Function  TreatAsAtomicUnit=on
  Switch : Switch  Threshold=3
  Steering Angle : Outport
  wires:
  Curvature/1 -> Driver Steering Model/1(Curvature)
  Longitudinal Velocity/1 -> Driver Steering Model/4(Longitudinal Velocity)
  Yaw Angle/1 -> Driver Steering Model/3(Yaw Angle)
  Lateral Velocity/1 -> Driver Steering Model/2(Lateral Velocity)
  Driver Steering Model/1(steering_ACC) -> Saturation/1
  turn_flag/1 -> Steering Angle for curve lane changing and u-turn/1(turn_flag), Switch/2
  Steering Angle for curve lane changing and u-turn/1(steering_curve_lane_changing_u_turn) -> Switch/1
  Switch/1 -> Steering Angle/1
  Saturation/1 -> Switch/3

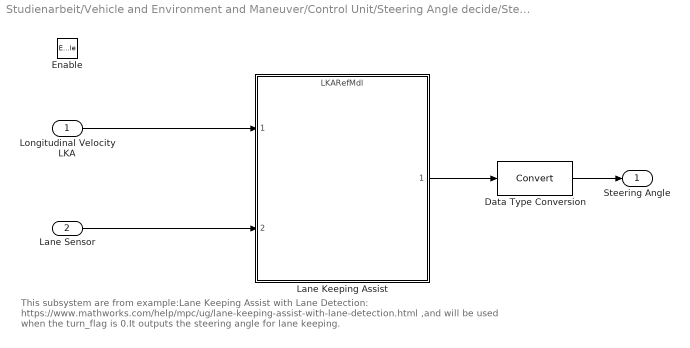
== system Studienarbeit/Vehicle and Environment and Maneuver/Control Unit/Steering Angle decide/Steering Angle LKA ==
  note: This subsystem are from example:Lane Keeping Assist with Lane Detection:
      | https://www.mathworks.com/help/mpc/ug/lane-keeping-assist-with-lane-detection.html ,and will be used when the turn_flag is 0.It outputs the steering angle for lane keeping.
  Longitudinal Velocity LKA : Inport
  Lane Sensor : Inport  Port=2
  Enable : EnablePort
  Data Type Conversion : DataTypeConversion
  Lane Keeping Assist : ModelReference  ModelNameDialog=LKARefMdl.slx  SimulationMode=Normal  CodeInterface=Top model  ModelReferenceVersion=1.289
  Steering Angle : Outport
  wires:
  Lane Sensor/1 -> Lane Keeping Assist/2
  Longitudinal Velocity LKA/1 -> Lane Keeping Assist/1
  Lane Keeping Assist/1 -> Data Type Conversion/1
  Data Type Conversion/1 -> Steering Angle/1

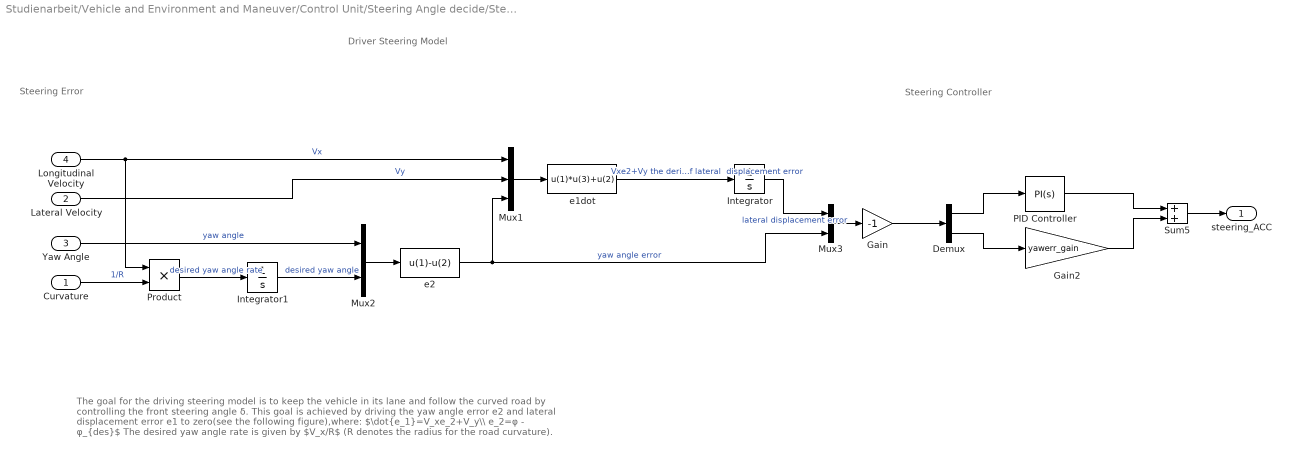
== system Studienarbeit/Vehicle and Environment and Maneuver/Control Unit/Steering Angle decide/Steering Angle /Driver Steering Model ==
  note: The goal for the driving steering model is to keep the vehicle in its lane and follow the curved road by controlling the front steering angle δ.
      | This goal is achieved by driving the yaw angle error e2 and lateral displacement error e1 to zero(see the following figure),where:
      | $\dot{e_1}=V_xe_2+V_y\\ e_2=φ - φ_{des}$
      | The desired yaw angle rate is given by $V_x/R$ (R denotes the radius for the road curvature).
  note: Steering Controller
  note: Steering Error
  note: Driver Steering Model
  Curvature : Inport
  Lateral Velocity : Inport  Port=2
  Yaw Angle : Inport  Port=3  Unit=rad
  Longitudinal Velocity : Inport  Port=4
  Demux : Demux  Outputs=2
  Gain : Gain  Gain=-1
  Gain2 : Gain  Gain=yawerr_gain
  Integrator : Integrator
  Integrator1 : Integrator
  Mux1 : Mux  Inputs=3
  Mux2 : Mux  Inputs=2
  Mux3 : Mux  Inputs=2
  PID Controller : simulink/Continuous/PID Controller  Controller=PI  Form=Parallel  TimeDomain=Continuous-time  UseExternalTs=off  SampleTime=-1  IntegratorMethod=Forward Euler  FilterMethod=Forward Euler  ControllerParametersSource=internal  P=driver_P  I=driver_I  D=0  UseFilter=on  N=100  TunerSelectOption=Transfer Function Based (PID Tuner App)  InitialConditionSource=internal  InitialConditionForIntegrator=0  InitialConditionForFilter=0  DifferentiatorICPrevScaledInput=0  ExternalReset=none  TrackingMode=off  Kt=1  LimitOutput=off  UpperSaturationLimit=inf  LowerSaturationLimit=-inf  LinearizeAsGain=on  AntiWindupMode=none  Kb=1  POutMin=[]  POutMax=[]  IOutMin=[]  IOutMax=[]  DOutMin=[]  DOutMax=[]  NOutMin=[]  NOutMax=[]  SumOutMin=[]  SumOutMax=[]  SaturationOutMin=[]  SaturationOutMax=[]  PParamMin=[]  PParamMax=[]  IParamMin=[]  IParamMax=[]  DParamMin=[]  DParamMax=[]  NParamMin=[]  NParamMax=[]  KbParamMin=[]  KbParamMax=[]  KtParamMin=[]  KtParamMax=[]  KbOutMin=[]  KbOutMax=[]  KtOutMin=[]  KtOutMax=[]  IntegratorOutMin=[]  IntegratorOutMax=[]  FilterOutMin=[]  FilterOutMax=[]  SumI1OutMin=[]  SumI1OutMax=[]  SumI2OutMin=[]  SumI2OutMax=[]  SumI3OutMin=[]  SumI3OutMax=[]  SumI4OutMin=[]  SumI4OutMax=[]  SumDOutMin=[]  SumDOutMax=[]  DifferentiatorOutMin=[]  DifferentiatorOutMax=[]  FilterDiffOutCoefMin=[]  FilterDiffOutCoefMax=[]  ReciprocalOutMin=[]  ReciprocalOutMax=[]  SumDenOutMin=[]  SumDenOutMax=[]  SumNumOutMin=[]  SumNumOutMax=[]  DivideOutMin=[]  DivideOutMax=[]  UdiffTsProdOutMin=[]  UdiffTsProdOutMax=[]  NTsProdOutMin=[]  NTsProdOutMax=[]  UintegralTsProdOutMin=[]  UintegralTsProdOutMax=[]  UngainTsProdOutMin=[]  UngainTsProdOutMax=[]  IntegratorContinuousStateAttributes=''  IntegratorStateMustResolveToSignalObject=off  IntegratorRTWStateStorageClass=Auto  FilterContinuousStateAttributes=''  FilterStateMustResolveToSignalObject=off  FilterRTWStateStorageClass=Auto  ParallelPVariant=InternalParameters  IdealPVariant=Disabled  IVariant=InternalParameters  DVariant=Disabled  IntegratorVariant=Continuous  SatVariant=Disabled  AWVariant=Passthrough  PCopyVariant=Disabled  TRVariant=Disabled  FdbkBlocksVariant=Forward  IdealPFdbkVariant=Disabled  SatFdbkVariant=Disabled  DerivativeFilterVariant=Disabled  NVariant=Disabled  NCopyVariant=Disabled_SignalSpec  FilterICVariant=Disabled  IntegratorICVariant=InternalICs  ExternalResetVariant=Disabled  TRSumVariant=Passthrough  SumFdbkVariant=Disabled  SumVariant=Sum_PI  TsampFilterVariant=InternalTs  TsampNgainVariant=Passthrough  TsampIntegralVariant=Passthrough
  Product : Product
  Sum5 : Sum
  e1dot : Fcn  Expr=u(1)*u(3)+u(2)
  e2 : Fcn  Expr=u(1)-u(2)
  steering_ACC : Outport  VectorParamsAs1DForOutWhenUnconnected=off
  wires:
  e1dot/1 -> Integrator/1  "Vxe2+Vy the derivative of lateral  displacement error"
  Mux2/1 -> e2/1
  e2/1 -> Mux3/2, Mux1/3  "yaw angle error"
  Mux3/1 -> Gain/1
  Lateral Velocity/1 -> Mux1/2  "Vy"
  Mux1/1 -> e1dot/1
  Integrator/1 -> Mux3/1  "lateral displacement error"
  Product/1 -> Integrator1/1  "desired yaw angle rate"
  Integrator1/1 -> Mux2/2  "desired yaw angle"
  Curvature/1 -> Product/2  "1/R"
  Longitudinal Velocity/1 -> Product/1, Mux1/1  "Vx"
  Gain2/1 -> Sum5/2
  PID Controller/1 -> Sum5/1
  Demux/2 -> Gain2/1
  Sum5/1 -> steering_ACC/1
  Demux/1 -> PID Controller/1
  Gain/1 -> Demux/1
  Yaw Angle/1 -> Mux2/1  "yaw angle"

== matlab function Studienarbeit/Vehicle and Environment and Maneuver/Control Unit/Steering Angle decide/Steering Angle /Steering Angle for curve lane changing and u-turn ==
  data: turn_flag input; steering_curve_lane_changing_u_turn output
function steering_curve_lane_changing_u_turn= curve_lane_or_u_turn(turn_flag)

% This function outputs a certain steering angle with different turn_flag
% value.

% Input:
% turn_flag: a flag to indicate the vehicle's maneuver.

% Output:
% steering_curve_lane_changing_u_turn: steering angle for curve lane
% changing or u-turn.

if turn_flag == 3 
    % The vehicle will switch left in a curve lane with a steering angle
    % 0.1 rad.
    
    steering_curve_lane_changing_u_turn = 0.1;
elseif turn_flag==5
    % The vehicle will decelerate and then turn left,before left turning
    % the vehicle will go right a little bit with a very small steering
    % angle,here -0.0013,negative sign means right.
    
    steering_curve_lane_changing_u_turn = -0.0013;
elseif turn_flag == 6 || turn_flag == 9
    % For turn_flag = 6,the vehicle will turn left with a steering angle 
    % 0.5 rad,and then go backwards.
    % For turn_flag = 9,the vehicle will turn left after a adjustment left
    % turning.
    
    steering_curve_lane_changing_u_turn = 0.5;
elseif turn_flag == 7
    % The vehicle will go backwards with a turning.
    
    steering_curve_lane_changing_u_turn = -0.5;
elseif turn_flag == 8
    % The vehicle will make a adjustment left turn to make its velocity
    % larger than 0.
    
    steering_curve_lane_changing_u_turn = 0.1;
else
    % For turn_flag = 4.The vehicle will switch right in a curve lane with 
    % a steering angle -0.1 rad.
    
    steering_curve_lane_changing_u_turn = -0.1;
end

== matlab function Studienarbeit/Vehicle and Environment and Maneuver/Control Unit/MIO Track/Pack MIO Track ==
  data: tracks input; mioTrack output Bus: BusMultiObjectTracker1; mioTrackIndex input
function mioTrack = fcn(tracks, mioTrackIndex)
% Extract MIO track and package for visualization in Birds Eye Scope

mioTrack = tracks;

if mioTrackIndex > 0
    % First track represents MIO
    mioTrack.NumTracks = 1;
    mioTrack.Tracks(1) = tracks.Tracks(mioTrackIndex);
else
    % No valid MIO track
    mioTrack.NumTracks = 0;
end

== matlab function Studienarbeit/Vehicle and Environment and Maneuver/Control Unit/Duration,Curvature and Longitudinal Acceleration calculation/Duration,Curvature and Acceleration calculation ==
  data: duration output; curvature output; d2x output; velocity_vehicle_B input; initial_lane_changing_velocity_ego input; t input; coor_trans_t input; turn_flag input; velocity_right_lane_max input; velocity_left_lane_max input; can_lane_changing output
function [duration,curvature,d2x,can_lane_changing]= getDurationandCurvatureandAcceleration(velocity_vehicle_B, initial_lane_changing_velocity_ego, t,coor_trans_t, turn_flag,velocity_right_lane_max,velocity_left_lane_max)
% Calculate the desired curvature,longitudinal velocity and duration of lane
% changing and u-turn maneuver.

% Inputs:
% velocity_vehicle_B: speed of the overtaken vehicle B. Unit: m/s
% safety_distance: safety distance between the projection of the
% vehicle A on its lane and the position of the vehicle B on that 
% lane, when A reaches ist lane;or the distance between vehicle ego 
% and B when ego vehicle finished the returning maneuver.
% initial_lane_changing_velocity_ego: the initial speed of lane changing maneuver.
% coor_trans_t: the start time of lane changing maneuver,which is
% used for coordinate transformation.
% turn_flag: 0->lane keeping,1,2->straight lane changing,3,4->curve lane
% changing,5,6,7,8->left u-turn
% velocity_right_lane_max: maximal speed allowed on the right lane.
% velocity_left_lane_max: maximal speed allowed on the left lane.

% Outputs:
% curvature: the desired curvature of lane changing.
% d2x: the desired longitudinal acceleration of lane changing.
% duration: the duration of lane changing or u-turn maneuver.
% can_lane_changing: 1->lane changing allowed;0->lane changing not allowed.

can_lane_changing=1; % the value will be set to one until a good condition for lane change is found.
% lateral_acceleration_max = 4; % maximal lateral acceleration
% lateral_acceleration_min = -4;% minimal lateral acceleration
% longitudinal_acceleration_max = 2; % maximal longitudinal acceleration
% longitudinal_acceleration_min = -2; % minimal longitudinal acceleration
% maximum speed allowed on the left/right lane. Unit:m/s.

% U-Turn:
% The main idea is to control the value of steering angle and acceleration,
% which are inputs for Vehicle Dynamics block.The Curvature has nothing to 
% do with u-turn so the value will all be zero.This part is about
% acceleration.
if turn_flag == 5
    % Deceleration: the vehicle will decelerate with a -2m/s^2 acceleration
    % to velocity about 0.3m/s,which will make the vehicle very slow while 
    % turning. The duration is given by: v_end = v_start + acceleration*t
    d2x = -2; 
    curvature = 0;
    duration= (0.3-initial_lane_changing_velocity_ego)/d2x;
elseif  turn_flag == 6
    % Turn left: the vehicle will turn left to arrive at the left lane,the
    % heading of the vehicle is not parallel to the left lane.The vehicle 
    % will then go backwards to make another left turn to finish u-turn.
    % The vehicle's velocity remains the same while turning left(d2x=0), the
    % duration is not calculated but from testing.
    d2x = 0;
    curvature = 0;
    duration= 10.5;
elseif turn_flag == 7
    % Backwards: the vehicle will go backwards to make another left
    % turning.In order to make the vehicle go backwards,the front and rear 
    % force of the bicycle model should be negative,according to the 
    % newton's second law: Force = mass*acceleration,the acceleration should
    % also be negative(d2x=-0.6).The duration is also from testing.
    d2x = -0.6;
    curvature = 0;
    duration= 4.9;
elseif turn_flag == 8
    % Adjustment turn left: after the backwards the velocity of the vehicle
    % will be negative,this will cause an error from Lane Keeping Controller
    %(the input longtitudinal velocity of the Lane Keeping controller
    % should be positive).Set the acceleration to a positive number to make
    % the velocity positive.The duration is also from testing.
    d2x = 2;
    curvature = 0;
    duration= 2;
elseif turn_flag == 9
    % Turn left: the vehicle will turn left with a constant velocity to 
    % arrive at the center of the left lane.The duration is also from testing. 
    d2x = 0;
    curvature = 0;
    duration= 6;

% Lane change
elseif turn_flag == 1|| turn_flag == 2    
    % turn_flag = 1:switch left
    % turn_flag = 2:switch right
    velocity_lane_max =  velocity_left_lane_max;
    if turn_flag == 2
    velocity_lane_max = velocity_right_lane_max; 
    end

    % straight lane change
    
    % the target speed velocity_ego_target should be greater than the overtaken
    % vehicle speed by at least 20km/h, while respecting the maximum speed 
    % allowed on the left lane, which yields: 
    % velocity_ego_target = min(velocity_vehicle_B+20km/h,velocity_left_lane_max)
    % velocity_leftlane_max is the maximum speed allowed on the left lane.
    % the vehicle A can not overtake the vehicle B unless its speed is greater 
    % than or equal to the overtaken vehicle speed,this yields: 
    % velocity_ego_target = max(min(velocity_vehicle_B+20km/h,velocity_left_lane_max),velocity_ego_initial)
    % https://tel.archives-ouvertes.fr/tel-01727720/file/These_UTC_Alia_Chebly.pdf,page 40,formula (2.32);
    velocity_ego_target=max(min(velocity_vehicle_B + 20*1000/3600, velocity_lane_max), initial_lane_changing_velocity_ego);
    distance_between_ego_B_initial = 20; %the distance between the ego vehicle 
    % and the overtaken vehicle at the beginning of the lane changing maneuver
    safety_distance = 3; % safety_distance: safety distance between the projection 
    % of the vehicle A on its lane and the position of the vehicle B on that 
    % lane, when A reaches ist lane;or the distance between vehicle ego 
    % and B when ego vehicle finished the returning maneuver.
    lane_width=3.6;%lane_width   

    % The derive of duration is at page 40,41,part:
    % Respecting safety requirements,formula (2.36)
    % https://tel.archives-ouvertes.fr/tel-01727720/file/These_UTC_Alia_Chebly.pdf

    duration = 2*(distance_between_ego_B_initial - safety_distance )/(velocity_ego_target + initial_lane_changing_velocity_ego - 2*velocity_vehicle_B);

    % https://tel.archives-ouvertes.fr/tel-01727720/file/These_UTC_Alia_Chebly.pdf
    % The derive of duration_lane_changing_min is at page 39,40,part:
    % Respecting the vehicle dynamic constraints,formula (2.25), (2.30)
    %duration_lane_changing_min_1 = max(sqrt(5.77*lane_width/lateral_acceleration_max), sqrt(-5.77*lane_width/lateral_acceleration_min));
    %duration_lane_changing_min_2 = (velocity_ego_target - initial_lane_changing_velocity_ego)/(2/3*longitudinal_acceleration_max);

    % page 41, formula(2.39)
    % In order to find a proper duration(the solution space is not empty),the 
    % minimal duration must less than the maximal duration.If the solution
    % space is empty,we decide not to change lane.
    % if max(duration_lane_changing_min_1,duration_lane_changing_min_2) < duration_lane_changing_max
    %     can_lane_changing = 1;
    % else
    %     can_lane_changing = 0;
    % end

    t = t - coor_trans_t; % coordinate transformation
    % the equation for longitudinal position:
    % x = a0 + a1*t + a2*t^2 + a3*t^3 + a4*t^4
    % https://tel.archives-ouvertes.fr/tel-01727720/file/These_UTC_Alia_Chebly.pdf
    % page 37,formula (2.15);page 38,formula (2.18)
    % a0 = 0;
    a1 = initial_lane_changing_velocity_ego;
    % a2 = 0;
    a3 = (velocity_ego_target - initial_lane_changing_velocity_ego)/duration^2;
    a4 = (-a3/(2*duration));

    % the equation for lateral position: 
    % y = b0 + b1*t + b2*t^2 + b3*t^3 + b4*t^4 + b5*t^5
    % https://tel.archives-ouvertes.fr/tel-01727720/file/These_UTC_Alia_Chebly.pdf
    % page 37,formula (2.16);page 38,formula (2.20)
    % b0 = 0;
    % b1 = 0;
    % b2 = 0;
    b3 = ((-1)^(turn_flag + 1))*10*lane_width/duration^3;
    b4 = ((-1)^(turn_flag + 1))*(-15)*lane_width/duration^4;
    b5 = ((-1)^(turn_flag + 1))*6*lane_width/duration^5;

    % Desired x position
    % x = a1*(time)+a3*(time)^3+a4*(time)^4;
    % Desired y position
    % y = b3*(time)^3+b4*(time)^4+b5*(time)^5;

    % Desired curvature;
    % https://en.wikipedia.org/wiki/Curvature
    % part:In terms of a general parametrization
    dx = a1 + 3*a3*t^2 + 4*a4*t^3 ; % longitudinal velocity 
    d2x= 6*a3*t + 12*a4*t^2; % longitudinal acceleration 
    dy = 3*b3*t^2 + 4*b4*t^3 + 5*b5*t^4; % lateral velocity 
    d2y = 6*b3*t + 12*b4*t^2 + 20*b5*t^3; % lateral acceleration 
    curvature = (dx*d2y - d2x*dy)/(dx^2 + dy^2)^(3/2); 

else
    d2x = 0;
    curvature=0;
    duration=0;
end

== stateflow chart Studienarbeit/Command ==
  note: initial_lane = 0: right lane
      | initial_lane = 1: left lane
      | current_lane = 0: right lane
      | current_lane = 1: left lane
      | lead_car = 1: there is a lead car
      | lead_car = 0: there is no lead car
      | man_or_auto = 0: manual mode
      | man_or_auto = 1: autonomous mode
      | lane_changed = 1: the vehicle changed its lane after it starts to run.
      | lane_changed = 0: the vehicle hasn't changed its lane after it starts to run.
  state autonomous_mode
    state switch_left_lead_car
      entry:
      command = 1;
      lane_changed = 1;
    state go_straight_after_switch_left
      entry:
      command=0;
    state go_straight_before_switch_right
      entry:
      command=0;
    state switch_right_after_switch_left
      entry:
      command = 2;
    state lane_keeping
      entry:
      command = 0;
    state switch_right_lead_car
      entry:
      command = 2;
      lane_changed = 1;
    state switch_left_after_switch_right
      entry:
      command = 1;
    state go_straight_after_switch_right
      entry:
      command=0;
    state go_straight_before_switch_left
      entry:
      command = 0;
    go_straight_after_switch_left -> go_straight_before_switch_right [order 1] : after(5,sec)[lead_car==0&&current_lane ==1]
    switch_left_lead_car -> go_straight_after_switch_left : after(1,sec)
    go_straight_before_switch_right -> switch_right_after_switch_left [order 2] : after(7,sec)
    switch_right_after_switch_left -> autonomous_mode.lane_keeping : after(1,sec)
    go_straight_before_switch_right -> autonomous_mode.lane_keeping [order 1] : [man_or_auto == 0]
    go_straight_before_switch_right -> autonomous_mode.lane_keeping [order 3] : after(5,sec)[curve_lane_or_not == 1]
    go_straight_after_switch_left -> autonomous_mode.lane_keeping [order 3] : [man_or_auto == 0]
    go_straight_after_switch_left -> autonomous_mode.lane_keeping [order 2] : after(5,sec)[lead_car == 1]
    go_straight_after_switch_left -> autonomous_mode.lane_keeping [order 4] : after(5,sec)[curve_lane_or_not == 1]
    autonomous_mode.lane_keeping -> switch_left_lead_car [order 2] : after(5,sec)[curve_lane_or_not ==0&&lead_car ==1&&consider_lane_changing==1&&can_lane_changing==1&&( current_lane ==0||(lane_changed == 0&&initial_lane==0))]
    (default) -> autonomous_mode.lane_keeping
    switch_left_after_switch_right -> autonomous_mode.lane_keeping : after(1,sec)
    go_straight_before_switch_left -> autonomous_mode.lane_keeping [order 1] : [man_or_auto==0]
    go_straight_before_switch_left -> autonomous_mode.lane_keeping [order 3] : after(5,sec)[curve_lane_or_not == 1]
    autonomous_mode.lane_keeping -> switch_right_lead_car [order 1] : after(5,sec)[curve_lane_or_not==0&&lead_car == 1&&consider_lane_changing==1 &&can_lane_changing==1&&( current_lane ==1||(lane_changed==0&&initial_lane==1))]
    go_straight_after_switch_right -> autonomous_mode.lane_keeping [order 3] : [man_or_auto == 0]
    go_straight_after_switch_right -> autonomous_mode.lane_keeping [order 2] : after(5,sec)[lead_car==1]
    go_straight_after_switch_right -> autonomous_mode.lane_keeping [order 4] : after(5,sec)[curve_lane_or_not == 1]
    go_straight_before_switch_left -> switch_left_after_switch_right [order 2] : after(7,sec)
    switch_right_lead_car -> go_straight_after_switch_right : after(1,sec)
    go_straight_after_switch_right -> go_straight_before_switch_left [order 1] : after(5,sec)[lead_car==0&& current_lane ==0]
  state manual_mode
    state switch_left_curve
      entry:
      command = 3;
    state lane_keeping
      entry:
      command = 0;
    state switch_left_straight
      entry:
      command = 1;
    state switch_right_straight
      entry:
      command = 2;
    state switch_right_curve
      entry:
      command=4;
    state Left_U_Turn
      entry:
      command = 5;
    (default) -> manual_mode.lane_keeping
    switch_left_curve -> manual_mode.lane_keeping : [command_manual == 0]
    switch_left_straight -> manual_mode.lane_keeping : [command_manual==0]
    manual_mode.lane_keeping -> switch_left_curve [order 3] : [command_manual == 1&&curve_lane_or_not == 1]
    manual_mode.lane_keeping -> switch_left_straight [order 1] : [command_manual == 1&&curve_lane_or_not == 0]
    manual_mode.lane_keeping -> switch_right_curve [order 4] : [command_manual == 2&&curve_lane_or_not == 1]
    manual_mode.lane_keeping -> switch_right_straight [order 2] : [command_manual == 2&&curve_lane_or_not == 0]
    switch_right_curve -> manual_mode.lane_keeping : [command_manual == 0]
    switch_right_straight -> manual_mode.lane_keeping : [command_manual == 0]
    manual_mode.lane_keeping -> Left_U_Turn [order 5] : [command_manual == 3]
    Left_U_Turn -> manual_mode.lane_keeping : [command_manual == 0]
  (default) -> autonomous_mode
  autonomous_mode -> manual_mode : [man_or_auto == 0]
  manual_mode -> autonomous_mode : [man_or_auto==1]
  data: can_lane_changing input; man_or_auto input; command output; consider_lane_changing input; lead_car input; command_manual input; initial_lane input; current_lane input; lane_changed local =0; curve_lane_or_not input
